simulink model "P4_ffilter"  (R2020b)
settings: Solver=VariableStepAuto  StartTime=0.0  StopTime=10.0  RelTol=1e-3
model workspace (MAT data in the model file):
  a1 = 0.5
  a2 = -0.25
  b1 = 0.4
  bo = 1
libraries: simulink x1
settings Model: Creator=mluser  LastModifiedBy=mluser

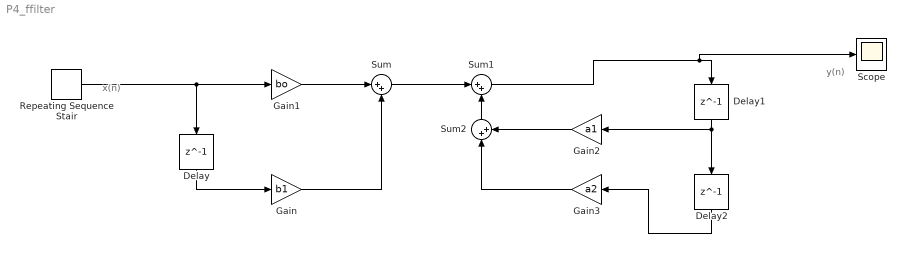
== system P4_ffilter ==
  note: y(n)
  note: x(n)
  Delay : Delay  DelayLength=1
  Delay1 : Delay  DelayLength=1
  Delay2 : Delay  DelayLength=1
  Gain : Gain  Gain=b1
  Gain1 : Gain  Gain=bo
  Gain2 : Gain  Gain=a1
  Gain3 : Gain  Gain=a2
  Repeating Sequence Stair : simulink/Sources/Repeating Sequence Stair  OutValues=[3 1 4 2 1].'  tsamp=-1  OutMin=[]  OutMax=[]  OutDataTypeStr=double  OutputDataTypeScalingMode=double  OutDataType=fixdt(0,8)  ConRadixGroup=Best Precision: Vector-wise  OutScaling=2^-12
  Scope : Scope
  Sum : Sum  Inputs=|++
  Sum1 : Sum  Inputs=|++
  Sum2 : Sum  Inputs=|++
  wires:
  Repeating Sequence Stair/1 -> Delay/1, Gain1/1
  Delay/1 -> Gain/1
  Gain1/1 -> Sum/1
  Gain/1 -> Sum/2
  Sum/1 -> Sum1/1
  Sum2/1 -> Sum1/2
  Gain2/1 -> Sum2/2
  Gain3/1 -> Sum2/1
  Delay1/1 -> Delay2/1, Gain2/1
  Delay2/1 -> Gain3/1
  Sum1/1 -> Scope/1, Delay1/1
